simulink model "exampleThermalNode"  (Simulink 7.6)
settings: Solver=ode45  StartTime=0.0  StopTime=2*3600  RelTol=1e-3
settings Model: Creator=drhf  LastModifiedBy=drhf

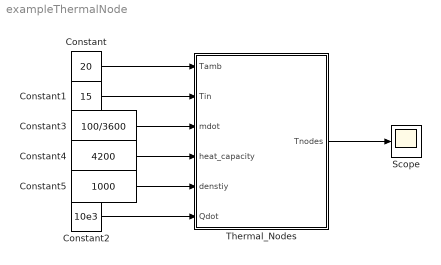
== system exampleThermalNode ==
  Constant : Constant  Value=20
  Constant1 : Constant  Value=15
  Constant2 : Constant  Value=10e3
  Constant3 : Constant  Value=100/3600
  Constant4 : Constant  Value=4200
  Constant5 : Constant  Value=1000
  Scope : Scope
  Thermal_Nodes : Subsystem
  wires:
  Thermal_Nodes/1(Tnodes) -> Scope/1
  Constant/1 -> Thermal_Nodes/1(Tamb)
  Constant1/1 -> Thermal_Nodes/2(Tin)
  Constant2/1 -> Thermal_Nodes/6(Qdot)
  Constant3/1 -> Thermal_Nodes/3(mdot)
  Constant4/1 -> Thermal_Nodes/4(heat_capacity)
  Constant5/1 -> Thermal_Nodes/5(denstiy)

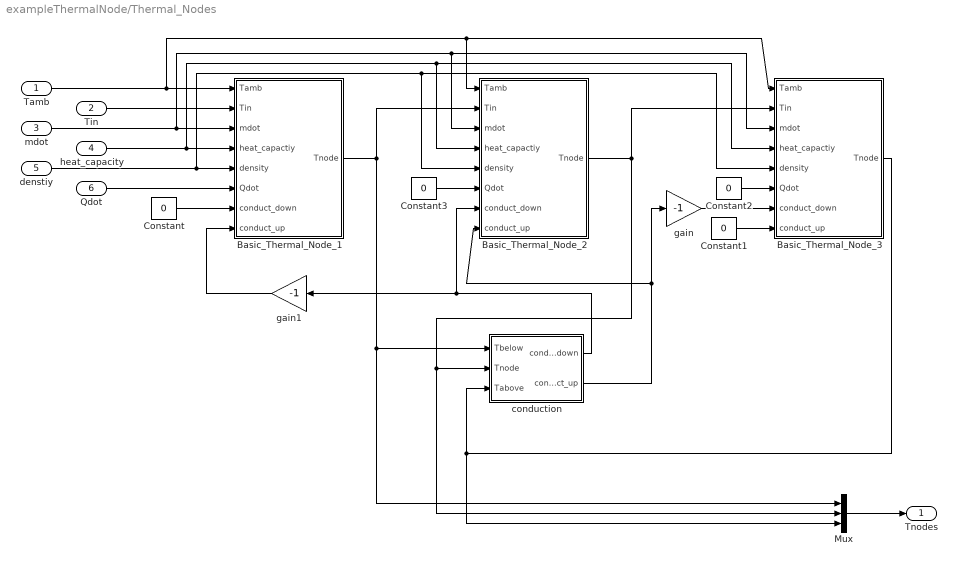
== system exampleThermalNode/Thermal_Nodes ==
  Tamb : Inport
  Tin : Inport  Port=2
  mdot : Inport  Port=3
  heat_capacity : Inport  Port=4
  denstiy : Inport  Port=5
  Qdot : Inport  Port=6
  Basic_Thermal_Node_1 : Subsystem  mask{Vnode=0.07, UA=1, Tinit=20}
      mask prompts: Vnode "Node volume in m³"; UA "Loss coefficient in W/K"; Tinit "Initial temperature in °C"
  Basic_Thermal_Node_2 : Subsystem  mask{Vnode=0.07, UA=1, Tinit=20}
      mask prompts: Vnode "Node volume in m³"; UA "Loss coefficient in W/K"; Tinit "Initial temperature in °C"
  Basic_Thermal_Node_3 : Subsystem  mask{Vnode=0.07, UA=1, Tinit=20}
      mask prompts: Vnode "Node volume in m³"; UA "Loss coefficient in W/K"; Tinit "Initial temperature in °C"
  Constant{,1..3} (4 alike) : Constant  Value=0
  Mux : Mux  Inputs=3
  conduction : Subsystem  mask{cond=1, d_below=0.5, d_above=0.5, convect=10}
      mask prompts: cond "conductivity"; d_below "distance to lower node"; d_above "distance to upper node"; convect "convective transport to upper node during thermal inversion"
  gain : Gain  Gain=-1  SaturateOnIntegerOverflow=on  OutDataTypeStr=Inherit: Same as input  ParamDataTypeStr=Inherit: Same as input
  gain1 : Gain  Gain=-1  SaturateOnIntegerOverflow=on  OutDataTypeStr=Inherit: Same as input  ParamDataTypeStr=Inherit: Same as input
  Tnodes : Outport
  wires:
  Basic_Thermal_Node_1/1(Tnode) -> conduction/1(Tbelow), Mux/1, Basic_Thermal_Node_2/2(Tin)
  Tamb/1 -> Basic_Thermal_Node_1/1(Tamb), Basic_Thermal_Node_2/1(Tamb), Basic_Thermal_Node_3/1(Tamb)
  Tin/1 -> Basic_Thermal_Node_1/2(Tin)
  mdot/1 -> Basic_Thermal_Node_1/3(mdot), Basic_Thermal_Node_2/3(mdot), Basic_Thermal_Node_3/3(mdot)
  heat_capacity/1 -> Basic_Thermal_Node_1/4(heat_capactiy), Basic_Thermal_Node_2/4(heat_capactiy), Basic_Thermal_Node_3/4(heat_capactiy)
  denstiy/1 -> Basic_Thermal_Node_1/5(density), Basic_Thermal_Node_2/5(density), Basic_Thermal_Node_3/5(density)
  Qdot/1 -> Basic_Thermal_Node_1/6(Qdot)
  Constant/1 -> Basic_Thermal_Node_1/7(conduct_down)
  Constant1/1 -> Basic_Thermal_Node_3/8(conduct_up)
  Basic_Thermal_Node_2/1(Tnode) -> conduction/2(Tnode), Mux/2, Basic_Thermal_Node_3/2(Tin)
  conduction/2(conduct_up) -> gain/1, Basic_Thermal_Node_2/8(conduct_up)
  gain/1 -> Basic_Thermal_Node_3/7(conduct_down)
  conduction/1(conduct_down) -> gain1/1, Basic_Thermal_Node_2/7(conduct_down)
  Basic_Thermal_Node_3/1(Tnode) -> conduction/3(Tabove), Mux/3
  gain1/1 -> Basic_Thermal_Node_1/8(conduct_up)
  Constant2/1 -> Basic_Thermal_Node_3/6(Qdot)
  Constant3/1 -> Basic_Thermal_Node_2/6(Qdot)
  Mux/1 -> Tnodes/1

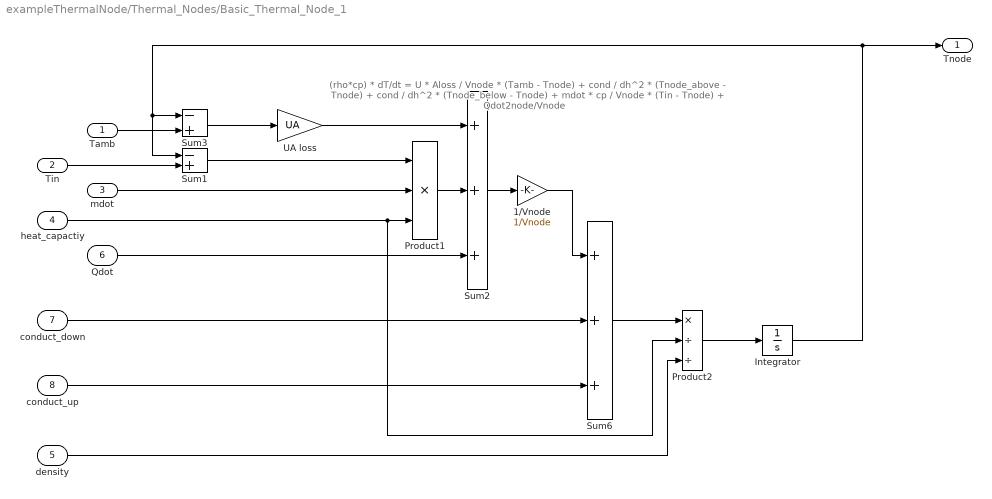
== system exampleThermalNode/Thermal_Nodes/Basic_Thermal_Node_1 ==
  note: (rho*cp) * dT/dt = U * Aloss / Vnode *      (Tamb        - Tnode)
      |                   + cond / dh^2 *            (Tnode_above - Tnode)
      |                   + cond / dh^2 *            (Tnode_below - Tnode)
      |                   + mdot * cp / Vnode *   (Tin         - Tnode)
      |                   + Qdot2node/Vnode
  Tamb : Inport
  Tin : Inport  Port=2
  mdot : Inport  Port=3
  heat_capactiy : Inport  Port=4
  density : Inport  Port=5
  Qdot : Inport  Port=6
  conduct_down : Inport  Port=7
  conduct_up : Inport  Port=8
  1/Vnode : Gain  Gain=1/Vnode  SaturateOnIntegerOverflow=on  OutDataTypeStr=Inherit: Same as input  ParamDataTypeStr=Inherit: Same as input
  Integrator : Integrator  InitialCondition=Tinit
  Product1 : Product  Inputs=3  SaturateOnIntegerOverflow=on  InputSameDT=on  OutDataTypeStr=Inherit: Same as first input
  Product2 : Product  Inputs=*//  SaturateOnIntegerOverflow=on  InputSameDT=on  OutDataTypeStr=Inherit: Same as first input
  Sum1 : Sum  Inputs=-+  SaturateOnIntegerOverflow=on  InputSameDT=on  OutDataTypeStr=Inherit: Same as first input
  Sum2 : Sum  Inputs=3  SaturateOnIntegerOverflow=on  InputSameDT=on  OutDataTypeStr=Inherit: Same as first input
  Sum3 : Sum  Inputs=-+  SaturateOnIntegerOverflow=on  InputSameDT=on  OutDataTypeStr=Inherit: Same as first input
  Sum6 : Sum  Inputs=3  SaturateOnIntegerOverflow=on  InputSameDT=on  OutDataTypeStr=Inherit: Same as first input
  UA loss : Gain  Gain=UA  SaturateOnIntegerOverflow=on  OutDataTypeStr=Inherit: Same as input  ParamDataTypeStr=Inherit: Same as input
  Tnode : Outport
  wires:
  Sum1/1 -> Product1/1
  heat_capactiy/1 -> Product1/3, Product2/2
  Sum3/1 -> UA loss/1
  UA loss/1 -> Sum2/1
  Tamb/1 -> Sum3/2
  Tin/1 -> Sum1/2
  mdot/1 -> Product1/2
  Product1/1 -> Sum2/2
  Integrator/1 -> Tnode/1, Sum3/1, Sum1/1
  Product2/1 -> Integrator/1
  density/1 -> Product2/3
  Qdot/1 -> Sum2/3
  conduct_down/1 -> Sum6/2
  conduct_up/1 -> Sum6/3
  Sum6/1 -> Product2/1
  Sum2/1 -> 1/Vnode/1
  1/Vnode/1 -> Sum6/1

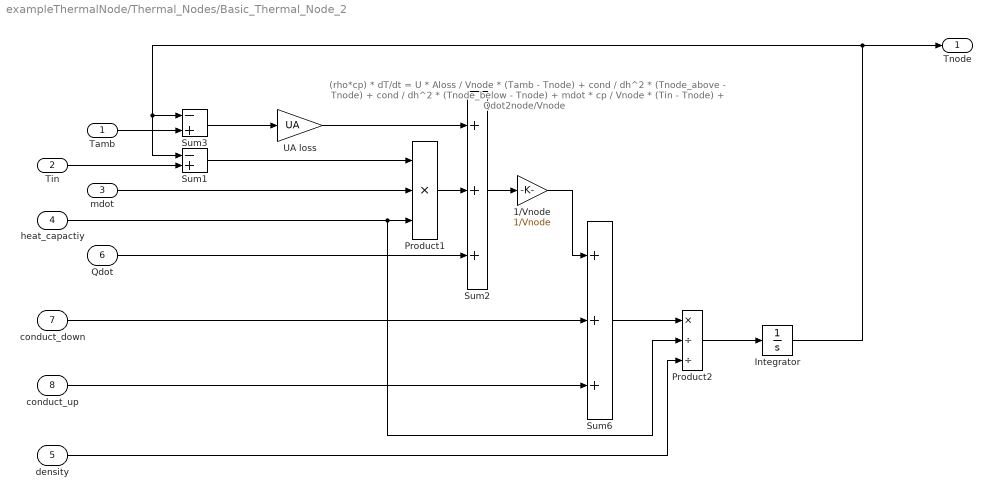
== system exampleThermalNode/Thermal_Nodes/Basic_Thermal_Node_2 ==
  note: (rho*cp) * dT/dt = U * Aloss / Vnode *      (Tamb        - Tnode)
      |                   + cond / dh^2 *            (Tnode_above - Tnode)
      |                   + cond / dh^2 *            (Tnode_below - Tnode)
      |                   + mdot * cp / Vnode *   (Tin         - Tnode)
      |                   + Qdot2node/Vnode
  Tamb : Inport
  Tin : Inport  Port=2
  mdot : Inport  Port=3
  heat_capactiy : Inport  Port=4
  density : Inport  Port=5
  Qdot : Inport  Port=6
  conduct_down : Inport  Port=7
  conduct_up : Inport  Port=8
  1/Vnode : Gain  Gain=1/Vnode  SaturateOnIntegerOverflow=on  OutDataTypeStr=Inherit: Same as input  ParamDataTypeStr=Inherit: Same as input
  Integrator : Integrator  InitialCondition=Tinit
  Product1 : Product  Inputs=3  SaturateOnIntegerOverflow=on  InputSameDT=on  OutDataTypeStr=Inherit: Same as first input
  Product2 : Product  Inputs=*//  SaturateOnIntegerOverflow=on  InputSameDT=on  OutDataTypeStr=Inherit: Same as first input
  Sum1 : Sum  Inputs=-+  SaturateOnIntegerOverflow=on  InputSameDT=on  OutDataTypeStr=Inherit: Same as first input
  Sum2 : Sum  Inputs=3  SaturateOnIntegerOverflow=on  InputSameDT=on  OutDataTypeStr=Inherit: Same as first input
  Sum3 : Sum  Inputs=-+  SaturateOnIntegerOverflow=on  InputSameDT=on  OutDataTypeStr=Inherit: Same as first input
  Sum6 : Sum  Inputs=3  SaturateOnIntegerOverflow=on  InputSameDT=on  OutDataTypeStr=Inherit: Same as first input
  UA loss : Gain  Gain=UA  SaturateOnIntegerOverflow=on  OutDataTypeStr=Inherit: Same as input  ParamDataTypeStr=Inherit: Same as input
  Tnode : Outport
  wires:
  1/Vnode/1 -> Sum6/1
  Sum2/1 -> 1/Vnode/1
  Sum6/1 -> Product2/1
  conduct_up/1 -> Sum6/3
  conduct_down/1 -> Sum6/2
  Qdot/1 -> Sum2/3
  density/1 -> Product2/3
  Product2/1 -> Integrator/1
  Integrator/1 -> Sum1/1, Sum3/1, Tnode/1
  Product1/1 -> Sum2/2
  mdot/1 -> Product1/2
  Tin/1 -> Sum1/2
  Tamb/1 -> Sum3/2
  UA loss/1 -> Sum2/1
  Sum3/1 -> UA loss/1
  heat_capactiy/1 -> Product2/2, Product1/3
  Sum1/1 -> Product1/1

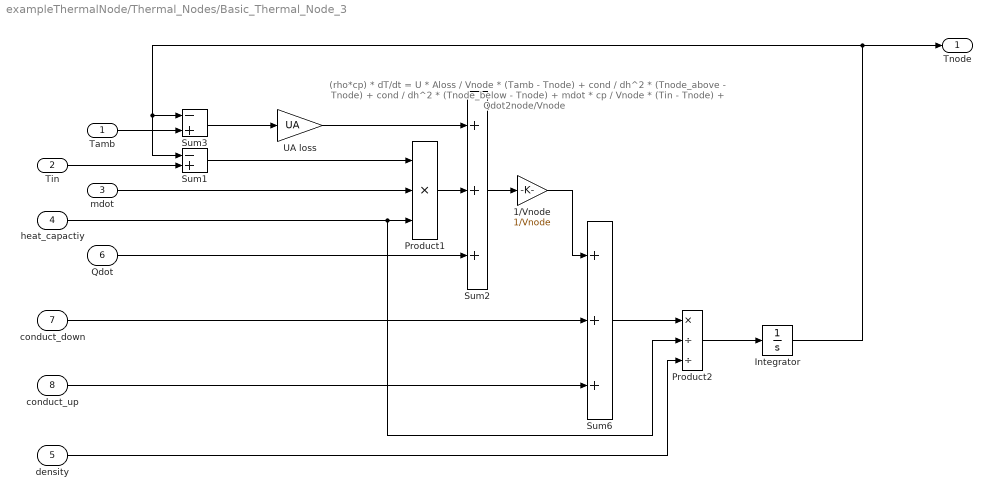
== system exampleThermalNode/Thermal_Nodes/Basic_Thermal_Node_3 ==
  note: (rho*cp) * dT/dt = U * Aloss / Vnode *      (Tamb        - Tnode)
      |                   + cond / dh^2 *            (Tnode_above - Tnode)
      |                   + cond / dh^2 *            (Tnode_below - Tnode)
      |                   + mdot * cp / Vnode *   (Tin         - Tnode)
      |                   + Qdot2node/Vnode
  Tamb : Inport
  Tin : Inport  Port=2
  mdot : Inport  Port=3
  heat_capactiy : Inport  Port=4
  density : Inport  Port=5
  Qdot : Inport  Port=6
  conduct_down : Inport  Port=7
  conduct_up : Inport  Port=8
  1/Vnode : Gain  Gain=1/Vnode  SaturateOnIntegerOverflow=on  OutDataTypeStr=Inherit: Same as input  ParamDataTypeStr=Inherit: Same as input
  Integrator : Integrator  InitialCondition=Tinit
  Product1 : Product  Inputs=3  SaturateOnIntegerOverflow=on  InputSameDT=on  OutDataTypeStr=Inherit: Same as first input
  Product2 : Product  Inputs=*//  SaturateOnIntegerOverflow=on  InputSameDT=on  OutDataTypeStr=Inherit: Same as first input
  Sum1 : Sum  Inputs=-+  SaturateOnIntegerOverflow=on  InputSameDT=on  OutDataTypeStr=Inherit: Same as first input
  Sum2 : Sum  Inputs=3  SaturateOnIntegerOverflow=on  InputSameDT=on  OutDataTypeStr=Inherit: Same as first input
  Sum3 : Sum  Inputs=-+  SaturateOnIntegerOverflow=on  InputSameDT=on  OutDataTypeStr=Inherit: Same as first input
  Sum6 : Sum  Inputs=3  SaturateOnIntegerOverflow=on  InputSameDT=on  OutDataTypeStr=Inherit: Same as first input
  UA loss : Gain  Gain=UA  SaturateOnIntegerOverflow=on  OutDataTypeStr=Inherit: Same as input  ParamDataTypeStr=Inherit: Same as input
  Tnode : Outport
  wires:
  Sum1/1 -> Product1/1
  heat_capactiy/1 -> Product1/3, Product2/2
  Sum3/1 -> UA loss/1
  UA loss/1 -> Sum2/1
  Tamb/1 -> Sum3/2
  Tin/1 -> Sum1/2
  mdot/1 -> Product1/2
  Product1/1 -> Sum2/2
  Integrator/1 -> Tnode/1, Sum3/1, Sum1/1
  Product2/1 -> Integrator/1
  density/1 -> Product2/3
  Qdot/1 -> Sum2/3
  conduct_down/1 -> Sum6/2
  conduct_up/1 -> Sum6/3
  Sum6/1 -> Product2/1
  Sum2/1 -> 1/Vnode/1
  1/Vnode/1 -> Sum6/1

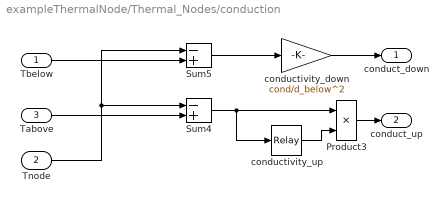
== system exampleThermalNode/Thermal_Nodes/conduction ==
  Tbelow : Inport
  Tnode : Inport  Port=2
  Tabove : Inport  Port=3
  Product3 : Product  SaturateOnIntegerOverflow=on  InputSameDT=on  OutDataTypeStr=Inherit: Same as first input
  Sum4 : Sum  Inputs=-+  SaturateOnIntegerOverflow=on  InputSameDT=on  OutDataTypeStr=Inherit: Same as first input
  Sum5 : Sum  Inputs=-+  SaturateOnIntegerOverflow=on  InputSameDT=on  OutDataTypeStr=Inherit: Same as first input
  conductivity_down : Gain  Gain=cond/d_below^2  SaturateOnIntegerOverflow=on  OutDataTypeStr=Inherit: Same as input  ParamDataTypeStr=Inherit: Same as input
  conductivity_up : Relay  OnSwitchValue=0  OffSwitchValue=-0.01  OnOutputValue=cond/d_above^2  OffOutputValue=convect*cond/d_above^2
  conduct_down : Outport
  conduct_up : Outport  Port=2
  wires:
  Sum5/1 -> conductivity_down/1
  Sum4/1 -> Product3/1, conductivity_up/1
  conductivity_up/1 -> Product3/2
  Tbelow/1 -> Sum5/2
  Tnode/1 -> Sum5/1, Sum4/1
  Tabove/1 -> Sum4/2
  conductivity_down/1 -> conduct_down/1
  Product3/1 -> conduct_up/1
